simulink model "sraam2023b"  (R2023b)
settings: Solver=ode4  StartTime=0.0  StopTime=25  FixedStep=0.001  RelTol=1e-3
values from neighbouring files (symbols this model uses):
  AEXIT = 0.0125    [SRAAM6_params.m]
  ALIMIT = 50.0    (= 50)    [SRAAM6_params.m]
  ALP_LIMX = 46.0    (= 46)    [SRAAM6_params.m]
  BIASAL = 0.0    (= 0)    [SRAAM6_params.m]
  DDLIMX = 600.0    (= 600)    [SRAAM6_params.m]
  DLIMX = 28.0    (= 28)    [SRAAM6_params.m]
  DPLIMX = 28.0    (= 28)    [SRAAM6_params.m]
  DQLIMX = 28.0    (= 28)    [SRAAM6_params.m]
  DRLIMX = 28.0    (= 28)    [SRAAM6_params.m]
  DT = 0.001    [SRAAM6_params.m]
  EBIASA = zeros(3,1)    [SRAAM6_params.m]
  EBIASG = zeros(3,1)    [SRAAM6_params.m]
  EMISA = zeros(3,1)    [SRAAM6_params.m]
  EMISG = zeros(3,1)    [SRAAM6_params.m]
  ESCALA = zeros(3,1)    [SRAAM6_params.m]
  ESCALG = zeros(3,1)    [SRAAM6_params.m]
  EUNBG = zeros(3,1)    [SRAAM6_params.m]
  FACT_WRCL = 0.0    (= 0)    [SRAAM6_params.m]
  GNAV = 4.0    (= 4)    [SRAAM6_params.m]
  INS_NOISE_PWR_A = 0.0    (= 0)    [SRAAM6_params.m]
  INS_NOISE_PWR_G = 0.0    (= 0)    [SRAAM6_params.m]
  K_ALPHA = 10.0    (= 10)    [SRAAM6_params.m]
  K_BETA = 10.0    (= 10)    [SRAAM6_params.m]
  MINS = 0    [SRAAM6_params.m]
  prop_cg_t = prop_cg_vs_time_t(:)    [SRAAM6_params.m]
  prop_cg_v = prop_cg_vs_time_v(:)    [SRAAM6_params.m]
  prop_mass_t = prop_mass_vs_time_t(:)    [SRAAM6_params.m]
  prop_mass_v = prop_mass_vs_time_v(:)    [SRAAM6_params.m]
  prop_moipitch_t = prop_moipitch_vs_time_t(:)    [SRAAM6_params.m]
  prop_moipitch_v = prop_moipitch_vs_time_v(:)    [SRAAM6_params.m]
  prop_moiroll_t = prop_moiroll_vs_time_t(:)    [SRAAM6_params.m]
  prop_moiroll_v = prop_moiroll_vs_time_v(:)    [SRAAM6_params.m]
  prop_thrust_t = prop_thrust_vs_time_t(:)    [SRAAM6_params.m]
  prop_thrust_v = prop_thrust_vs_time_v(:)    [SRAAM6_params.m]
  REFA = 0.01824    [SRAAM6_params.m]
  REFL = 0.1524    [SRAAM6_params.m]
  SCENARIO = 12    [SRAAM6_params.m]
  TGET_POS_IC = TGET_POS(SCENARIO, :)'    [SRAAM6_params.m]
  TGET_VEL_IC = TGET_VEL(SCENARIO, :)'    [SRAAM6_params.m]
  WBLIMX = 30.0    (= 30)    [SRAAM6_params.m]
  WN_NDI_Q = 50.0    (= 50)    [SRAAM6_params.m]
  WN_NDI_R = 50.0    (= 50)    [SRAAM6_params.m]
  WNACT = 251.0    (= 251)    [SRAAM6_params.m]
  X_IC = [SBEL_INIT; VBEB_IC; Q_IC; OMEGA_IC]    [SRAAM6_params.m]
  XCG_REF = 1.2994    [SRAAM6_params.m]
  ZETACT = 0.7    [SRAAM6_params.m]
  ZRCL = 0.9    [SRAAM6_params.m]
undefined symbols (not defined in the file or in its folder): alpha_bp, beta_bp, ca0_vs_mach, ca0b_vs_mach, caa_vs_mach_alpha_beta, cad_vs_mach, cll0_vs_mach_alpha_beta, clldp_vs_mach_alpha_beta, cllp_vs_mach, clm0_vs_mach_alpha_beta, clmdq_vs_mach_alpha_beta, clmq_vs_mach, cln0_vs_mach_alpha_beta, clndr_vs_mach_alpha_beta, clnr_vs_mach, cn0_vs_mach_alpha_beta, cndq_vs_mach_alpha_beta, cy0_vs_mach_alpha_beta, cydr_vs_mach_alpha_beta, mach_bp
libraries: simulink x3
(part 1 of 2)
settings Model: Creator=yagiz  LastModifiedBy=yagiz
settings DataIOCC: SaveFormat=Array  SaveState=on
settings RTWCC: GPUComputeCapability=5.0

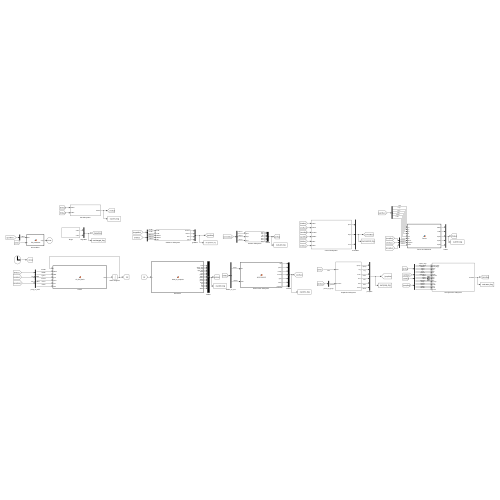
[thumbnail: Simulink's stored preview of the top-level diagram]
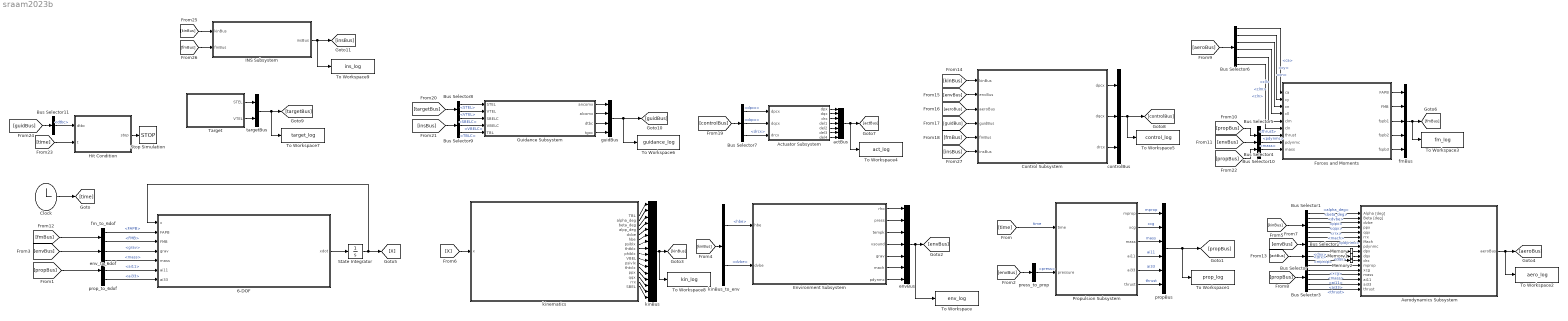
== system sraam2023b ==
  6-DOF : MATLAB Function  TreatAsAtomicUnit=on
  Actuator Subsystem : Subsystem
  Aerodynamics Subsystem : Subsystem
  Bus Selector : BusSelector  OutputSignals=dpx,dqx,drx
  Bus Selector1 : BusSelector  OutputSignals=alpha_deg,beta_deg,dvbe,ppx,qqx,rrx
  Bus Selector10 : BusSelector  OutputSignals=mass
  Bus Selector11 : BusSelector  OutputSignals=dtbc
  Bus Selector2 : BusSelector  OutputSignals=mach,pdynmc
  Bus Selector3 : BusSelector  OutputSignals=mprop,xcg,mass,ai11,ai33,thrust
  Bus Selector4 : BusSelector  OutputSignals=pdynmc
  Bus Selector5 : BusSelector  OutputSignals=thrust
  Bus Selector6 : BusSelector  OutputSignals=ca,cy,cn,cll,clm,cln
  Bus Selector7 : BusSelector  OutputSignals=dpcx,dqcx,drcx
  Bus Selector8 : BusSelector  OutputSignals=STEL,VTEL
  Bus Selector9 : BusSelector  OutputSignals=SBELC,VBELC,TBLC
  Clock : Clock
  Control Subsystem : Subsystem
  Environment Subsystem : MATLAB Function  TreatAsAtomicUnit=on
  Forces and Moments : MATLAB Function  TreatAsAtomicUnit=on
  Guidance Subsystem : Subsystem
  Hit Condition : MATLAB Function  TreatAsAtomicUnit=on
  INS Subsystem : Subsystem
  Memory : Memory
  Memory1 : Memory
  Memory2 : Memory
  Propulsion Subsystem : Subsystem
  State Integrator : Integrator  InitialCondition=X_IC
  Stop Simulation : Stop
  Target : Subsystem
  To Workspace : ToWorkspace  VariableName=env_log  SaveFormat=Timeseries  SampleTime=-1
  To Workspace1 : ToWorkspace  VariableName=prop_log  SaveFormat=Timeseries  SampleTime=-1
  To Workspace2 : ToWorkspace  VariableName=aero_log  SaveFormat=Timeseries  SampleTime=-1
  To Workspace3 : ToWorkspace  VariableName=fm_log  SaveFormat=Timeseries  SampleTime=-1
  To Workspace4 : ToWorkspace  VariableName=act_log  SaveFormat=Timeseries  SampleTime=-1
  To Workspace5 : ToWorkspace  VariableName=control_log  SaveFormat=Timeseries  SampleTime=-1
  To Workspace6 : ToWorkspace  VariableName=guidance_log  SaveFormat=Timeseries  SampleTime=-1
  To Workspace7 : ToWorkspace  VariableName=target_log  SaveFormat=Timeseries  SampleTime=-1
  To Workspace8 : ToWorkspace  VariableName=kin_log  SaveFormat=Timeseries  SampleTime=-1
  To Workspace9 : ToWorkspace  VariableName=ins_log  SaveFormat=Timeseries  SampleTime=-1
  actBus : BusCreator  Inputs=7
  controlBus : BusCreator  Inputs=3
  envBus : BusCreator  Inputs=7
  env_to_6dof : BusSelector  OutputSignals=grav
  fmBus : BusCreator  Inputs=5
  fm_to_6dof : BusSelector  OutputSignals=FAPB,FMB
  guidBus : BusCreator  Inputs=4
  kinBus : BusCreator  Inputs=16
  kinBus_to_env : BusSelector  OutputSignals=hbe,dvbe
  kinematics : MATLAB Function  TreatAsAtomicUnit=on
  press_to_prop : BusSelector  OutputSignals=press
  propBus : BusCreator  Inputs=6
  prop_to_6dof : BusSelector  OutputSignals=mass,ai11,ai33
  targetBus : BusCreator  Inputs=2
  wires:
  6-DOF/1(xdot) -> State Integrator/1
  State Integrator/1 -> [X], 6-DOF/1(x)
  Clock/1 -> [time]
  Environment Subsystem/7(pdynmc) -> envBus/7
  Environment Subsystem/6(mach) -> envBus/6
  Environment Subsystem/5(grav) -> envBus/5
  Environment Subsystem/4(vsound) -> envBus/4
  Environment Subsystem/3(tempk) -> envBus/3
  Environment Subsystem/2(press) -> envBus/2
  Environment Subsystem/1(rho) -> envBus/1
  envBus/1 -> To Workspace/1, [envBus]
  press_to_prop/1 -> Propulsion Subsystem/2(pressure)  "<press>"
  [time] -> Propulsion Subsystem/1(time)  "time"
  Propulsion Subsystem/1(mprop) -> propBus/1  "mprop"
  Propulsion Subsystem/2(xcg) -> propBus/2  "xcg"
  Propulsion Subsystem/3(mass) -> propBus/3  "mass"
  Propulsion Subsystem/4(ai11) -> propBus/4  "ai11"
  Propulsion Subsystem/5(ai33) -> propBus/5  "ai33"
  Propulsion Subsystem/6(thrust) -> propBus/6  "thrust"
  propBus/1 -> [propBus], To Workspace1/1
  [propBus] -> prop_to_6dof/1
  prop_to_6dof/1 -> 6-DOF/5(mass)  "<mass>"
  prop_to_6dof/2 -> 6-DOF/6(ai11)  "<ai11>"
  prop_to_6dof/3 -> 6-DOF/7(ai33)  "<ai33>"
  [envBus] -> press_to_prop/1
  [envBus] -> env_to_6dof/1
  env_to_6dof/1 -> 6-DOF/4(grav)  "<grav>"
  [X] -> kinematics/1(x)
  Aerodynamics Subsystem/1(aeroBus) -> To Workspace2/1, [aeroBus]
  kinematics/1(TBL) -> kinBus/1
  kinematics/2(alpha_deg) -> kinBus/2
  kinematics/3(beta_deg) -> kinBus/3
  kinematics/4(alpp_deg) -> kinBus/4
  kinematics/5(dvbe) -> kinBus/5
  kinematics/6(hbe) -> kinBus/6
  kinematics/7(psiblx) -> kinBus/7
  kinematics/8(thtblx) -> kinBus/8
  kinematics/9(phiblx) -> kinBus/9
  kinematics/10(VBEL) -> kinBus/10
  kinematics/11(psivlx) -> kinBus/11
  kinematics/12(thtvlx) -> kinBus/12
  kinBus/1 -> To Workspace8/1, [kinBus]
  [kinBus] -> kinBus_to_env/1
  kinBus_to_env/1 -> Environment Subsystem/1(hbe)  "<hbe>"
  kinBus_to_env/2 -> Environment Subsystem/2(dvbe)  "<dvbe>"
  [kinBus] -> Bus Selector1/1
  Bus Selector1/1 -> Aerodynamics Subsystem/1(Alpha [deg])  "<alpha_deg>"
  Bus Selector1/2 -> Aerodynamics Subsystem/2(Beta [deg])  "<beta_deg>"
  Bus Selector1/3 -> Aerodynamics Subsystem/3(dvbe)  "<dvbe>"
  Bus Selector1/4 -> Aerodynamics Subsystem/4(ppx)  "<ppx>"
  Bus Selector1/5 -> Aerodynamics Subsystem/5(qqx)  "<qqx>"
  Bus Selector1/6 -> Aerodynamics Subsystem/6(rrx)  "<rrx>"
  [envBus] -> Bus Selector2/1
  Bus Selector2/1 -> Aerodynamics Subsystem/7(Mach)  "<mach>"
  Bus Selector2/2 -> Aerodynamics Subsystem/8(pdynmc)  "<pdynmc>"
  [propBus] -> Bus Selector3/1
  Bus Selector3/1 -> Aerodynamics Subsystem/12(mprop)  "<mprop>"
  Bus Selector3/2 -> Aerodynamics Subsystem/13(xcg)  "<xcg>"
  Bus Selector3/3 -> Aerodynamics Subsystem/14(mass)  "<mass>"
  Bus Selector3/4 -> Aerodynamics Subsystem/15(ai11)  "<ai11>"
  Bus Selector3/5 -> Aerodynamics Subsystem/16(ai33)  "<ai33>"
  Bus Selector3/6 -> Aerodynamics Subsystem/17(thrust)  "<thrust>"
  [envBus] -> Bus Selector4/1
  Bus Selector4/1 -> Forces and Moments/8(pdynmc)  "<pdynmc>"
  [propBus] -> Bus Selector5/1
  [aeroBus] -> Bus Selector6/1
  Bus Selector6/1 -> Forces and Moments/1(ca)  "<ca>"
  Bus Selector6/2 -> Forces and Moments/2(cy)  "<cy>"
  Bus Selector6/3 -> Forces and Moments/3(cn)  "<cn>"
  Bus Selector6/4 -> Forces and Moments/4(cll)  "<cll>"
  Bus Selector6/5 -> Forces and Moments/5(clm)  "<clm>"
  Bus Selector6/6 -> Forces and Moments/6(cln)  "<cln>"
  Bus Selector5/1 -> Forces and Moments/7(thrust)  "<thrust>"
  Forces and Moments/1(FAPB) -> fmBus/1
  Forces and Moments/2(FMB) -> fmBus/2
  [fmBus] -> fm_to_6dof/1
  fm_to_6dof/1 -> 6-DOF/2(FAPB)  "<FAPB>"
  fm_to_6dof/2 -> 6-DOF/3(FMB)  "<FMB>"
  Actuator Subsystem/1(dpx) -> actBus/1
  Actuator Subsystem/2(dqx) -> actBus/2
  Actuator Subsystem/3(drx) -> actBus/3
  Actuator Subsystem/4(del1) -> actBus/4
  Actuator Subsystem/5(del2) -> actBus/5
  Actuator Subsystem/6(del3) -> actBus/6
  Actuator Subsystem/7(del4) -> actBus/7
  actBus/1 -> To Workspace4/1, [actBus]
  [actBus] -> Bus Selector/1
  Bus Selector/1 -> Memory/1  "<dpx>"
  Bus Selector/2 -> Memory1/1  "<dqx>"
  Bus Selector/3 -> Memory2/1  "<drx>"
  [kinBus] -> Control Subsystem/1(kinBus)
  [envBus] -> Control Subsystem/2(envBus)
  [aeroBus] -> Control Subsystem/3(aeroBus)
  controlBus/1 -> To Workspace5/1, [controlBus]
  [controlBus] -> Bus Selector7/1
  Bus Selector7/2 -> Actuator Subsystem/2(dqcx)  "<dqcx>"
  Bus Selector7/3 -> Actuator Subsystem/3(drcx)  "<drcx>"
  Bus Selector7/1 -> Actuator Subsystem/1(dpcx)  "<dpcx>"
  Control Subsystem/1(dpcx) -> controlBus/1
  Memory/1 -> Aerodynamics Subsystem/9(dpx)
  Memory1/1 -> Aerodynamics Subsystem/10(dqx)
  Memory2/1 -> Aerodynamics Subsystem/11(drx)
  Target/1(STEL) -> targetBus/1
  Target/2(VTEL) -> targetBus/2
  targetBus/1 -> To Workspace7/1, [targetBus]
  [targetBus] -> Bus Selector8/1
  Bus Selector8/1 -> Guidance Subsystem/1(STEL)  "<STEL>"
  Bus Selector8/2 -> Guidance Subsystem/2(VTEL)  "<VTEL>"
  [insBus] -> Bus Selector9/1
  Guidance Subsystem/1(ancomx) -> guidBus/1
  Guidance Subsystem/2(alcomx) -> guidBus/2
  guidBus/1 -> To Workspace6/1, [guidBus]
  [guidBus] -> Control Subsystem/4(guidBus)
  [propBus] -> Bus Selector10/1
  Bus Selector10/1 -> Forces and Moments/9(mass)  "<mass>"
  fmBus/1 -> [fmBus], To Workspace3/1
  [fmBus] -> Control Subsystem/5(fmBus)
  Guidance Subsystem/3(dtbc) -> guidBus/3
  Guidance Subsystem/4(tgoc) -> guidBus/4
  [time] -> Hit Condition/2(t)
  [guidBus] -> Bus Selector11/1
  Bus Selector11/1 -> Hit Condition/1(dtbc)  "<dtbc>"
  Hit Condition/1(stop) -> Stop Simulation/1
  Control Subsystem/2(dqcx) -> controlBus/2
  Control Subsystem/3(drcx) -> controlBus/3
  kinematics/13(ppx) -> kinBus/13
  kinematics/14(qqx) -> kinBus/14
  kinematics/15(rrx) -> kinBus/15
  kinematics/16(SBEL) -> kinBus/16
  Forces and Moments/3(fspb1) -> fmBus/3
  Forces and Moments/4(fspb2) -> fmBus/4
  Forces and Moments/5(fspb3) -> fmBus/5
  [kinBus] -> INS Subsystem/1(kinBus)
  [fmBus] -> INS Subsystem/2(fmBus)
  INS Subsystem/1(insBus) -> To Workspace9/1, [insBus]
  Bus Selector9/1 -> Guidance Subsystem/3(SBELC)  "<SBELC>"
  Bus Selector9/2 -> Guidance Subsystem/4(VBELC)  "<VBELC>"
  Bus Selector9/3 -> Guidance Subsystem/5(TBL)  "<TBLC>"
  [insBus] -> Control Subsystem/6(insBus)

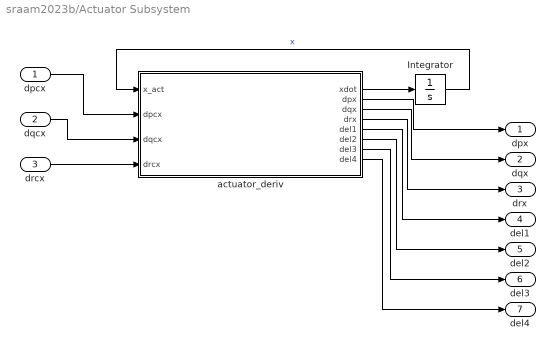
== system sraam2023b/Actuator Subsystem ==
  dpcx : Inport
  dqcx : Inport  Port=2
  drcx : Inport  Port=3
  Integrator : Integrator  InitialCondition=zeros(8, 1)
  actuator_deriv : MATLAB Function  TreatAsAtomicUnit=on
  dpx : Outport
  dqx : Outport  Port=2
  drx : Outport  Port=3
  del1 : Outport  Port=4
  del2 : Outport  Port=5
  del3 : Outport  Port=6
  del4 : Outport  Port=7
  wires:
  actuator_deriv/1(xdot) -> Integrator/1
  Integrator/1 -> actuator_deriv/1(x_act)  "x"
  dpcx/1 -> actuator_deriv/2(dpcx)
  dqcx/1 -> actuator_deriv/3(dqcx)
  drcx/1 -> actuator_deriv/4(drcx)
  actuator_deriv/2(dpx) -> dpx/1
  actuator_deriv/3(dqx) -> dqx/1
  actuator_deriv/4(drx) -> drx/1
  actuator_deriv/5(del1) -> del1/1
  actuator_deriv/6(del2) -> del2/1
  actuator_deriv/7(del3) -> del3/1
  actuator_deriv/8(del4) -> del4/1

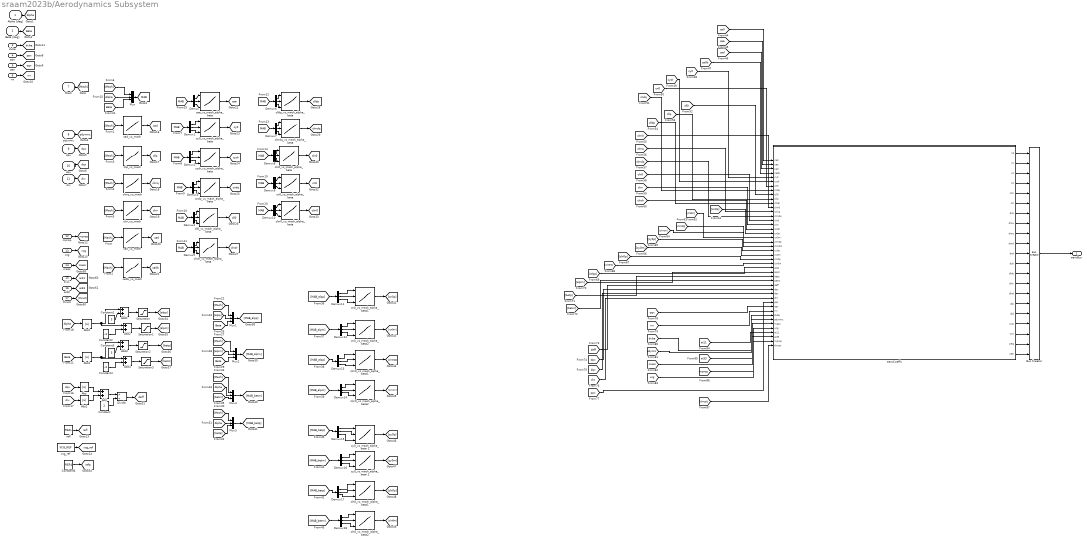
== system sraam2023b/Aerodynamics Subsystem ==
  Alpha [deg] : Inport
  Beta [deg] : Inport  Port=2
  dvbe : Inport  Port=3
  ppx : Inport  Port=4
  qqx : Inport  Port=5
  rrx : Inport  Port=6
  Mach : Inport  Port=7
  pdynmc : Inport  Port=8
  dpx : Inport  Port=9
  dqx : Inport  Port=10
  drx : Inport  Port=11
  mprop : Inport  Port=12
  xcg : Inport  Port=13
  mass : Inport  Port=14
  ai11 : Inport  Port=15
  ai33 : Inport  Port=16
  thrust : Inport  Port=17
  Abs{,1..3} (4 alike) : Abs  SaturateOnIntegerOverflow=off
  Add{,1..4} (5 alike) : Sum
  Bus Creator : BusCreator  Inputs=21
  Constant : Constant  Value=2
  Constant1 : Constant  Value=3
  Constant2 : Constant  Value=-3
  Constant3 : Constant  Value=3
  Constant4 : Constant  Value=-3
  Constant6 : Constant  Value=REFA
  Demux{,1..18} (19 alike) : Demux  Outputs=3
  Divide : Product  Inputs=*/
  Mux{,1..4} (5 alike) : Mux  Inputs=3
  Saturation : Saturate  UpperLimit=inf  LowerLimit=3
  Saturation1 : Saturate  UpperLimit=inf  LowerLimit=0
  Saturation2 : Saturate  UpperLimit=inf  LowerLimit=3
  Saturation3 : Saturate  UpperLimit=inf  LowerLimit=0
  aeroCoeffs : MATLAB Function  TreatAsAtomicUnit=on
  ca0_vs_mach : Lookup_n-D  NumberOfTableDimensions=1  BreakpointsForDimension1=mach_bp  Table=ca0_vs_mach  InternalRulePriority=Speed  RndMeth=Simplest
  ca0b_vs_mach : Lookup_n-D  NumberOfTableDimensions=1  BreakpointsForDimension1=mach_bp  Table=ca0b_vs_mach  InternalRulePriority=Speed  RndMeth=Simplest
  caa_vs_mach_alpha_beta : Lookup_n-D  NumberOfTableDimensions=3  BreakpointsForDimension1=mach_bp  BreakpointsForDimension2=alpha_bp  BreakpointsForDimension3=beta_bp  Table=caa_vs_mach_alpha_beta  InternalRulePriority=Speed  RndMeth=Simplest
      settings: InputPortMap=u0,u1,u2
  cad_vs_mach : Lookup_n-D  NumberOfTableDimensions=1  BreakpointsForDimension1=mach_bp  Table=cad_vs_mach  InternalRulePriority=Speed  RndMeth=Simplest
  cll0_vs_mach_alpha_beta : Lookup_n-D  NumberOfTableDimensions=3  BreakpointsForDimension1=mach_bp  BreakpointsForDimension2=alpha_bp  BreakpointsForDimension3=beta_bp  Table=cll0_vs_mach_alpha_beta  InternalRulePriority=Speed  RndMeth=Simplest
      settings: InputPortMap=u0,u1,u2
  clldp_vs_mach_alpha_beta : Lookup_n-D  NumberOfTableDimensions=3  BreakpointsForDimension1=mach_bp  BreakpointsForDimension2=alpha_bp  BreakpointsForDimension3=beta_bp  Table=clldp_vs_mach_alpha_beta  InternalRulePriority=Speed  RndMeth=Simplest
      settings: InputPortMap=u0,u1,u2
  cllp_vs_mach : Lookup_n-D  NumberOfTableDimensions=1  BreakpointsForDimension1=mach_bp  Table=cllp_vs_mach  InternalRulePriority=Speed  RndMeth=Simplest
  clm0_vs_mach_alpha_beta : Lookup_n-D  NumberOfTableDimensions=3  BreakpointsForDimension1=mach_bp  BreakpointsForDimension2=alpha_bp  BreakpointsForDimension3=beta_bp  Table=clm0_vs_mach_alpha_beta  InternalRulePriority=Speed  RndMeth=Simplest
      settings: InputPortMap=u0,u1,u2
  clm0_vs_mach_alpha_beta1 : Lookup_n-D  NumberOfTableDimensions=3  BreakpointsForDimension1=mach_bp  BreakpointsForDimension2=alpha_bp  BreakpointsForDimension3=beta_bp  Table=clm0_vs_mach_alpha_beta  InternalRulePriority=Speed  RndMeth=Simplest
      settings: InputPortMap=u0,u1,u2
  clm0_vs_mach_alpha_beta2 : Lookup_n-D  NumberOfTableDimensions=3  BreakpointsForDimension1=mach_bp  BreakpointsForDimension2=alpha_bp  BreakpointsForDimension3=beta_bp  Table=clm0_vs_mach_alpha_beta  InternalRulePriority=Speed  RndMeth=Simplest
      settings: InputPortMap=u0,u1,u2
  clmdq_vs_mach_alpha_beta : Lookup_n-D  NumberOfTableDimensions=3  BreakpointsForDimension1=mach_bp  BreakpointsForDimension2=alpha_bp  BreakpointsForDimension3=beta_bp  Table=clmdq_vs_mach_alpha_beta  InternalRulePriority=Speed  RndMeth=Simplest
      settings: InputPortMap=u0,u1,u2
  clmq_vs_mach : Lookup_n-D  NumberOfTableDimensions=1  BreakpointsForDimension1=mach_bp  Table=clmq_vs_mach  InternalRulePriority=Speed  RndMeth=Simplest
  cln0_vs_mach_alpha_beta : Lookup_n-D  NumberOfTableDimensions=3  BreakpointsForDimension1=mach_bp  BreakpointsForDimension2=alpha_bp  BreakpointsForDimension3=beta_bp  Table=cln0_vs_mach_alpha_beta  InternalRulePriority=Speed  RndMeth=Simplest
      settings: InputPortMap=u0,u1,u2
  cln0_vs_mach_alpha_beta1 : Lookup_n-D  NumberOfTableDimensions=3  BreakpointsForDimension1=mach_bp  BreakpointsForDimension2=alpha_bp  BreakpointsForDimension3=beta_bp  Table=cln0_vs_mach_alpha_beta  InternalRulePriority=Speed  RndMeth=Simplest
      settings: InputPortMap=u0,u1,u2
  cln0_vs_mach_alpha_beta2 : Lookup_n-D  NumberOfTableDimensions=3  BreakpointsForDimension1=mach_bp  BreakpointsForDimension2=alpha_bp  BreakpointsForDimension3=beta_bp  Table=cln0_vs_mach_alpha_beta  InternalRulePriority=Speed  RndMeth=Simplest
      settings: InputPortMap=u0,u1,u2
  "clndr_vs_mach_alpha_beta " : Lookup_n-D  NumberOfTableDimensions=3  BreakpointsForDimension1=mach_bp  BreakpointsForDimension2=alpha_bp  BreakpointsForDimension3=beta_bp  Table=clndr_vs_mach_alpha_beta  InternalRulePriority=Speed  RndMeth=Simplest
      settings: InputPortMap=u0,u1,u2
  clnr_vs_mach : Lookup_n-D  NumberOfTableDimensions=1  BreakpointsForDimension1=mach_bp  Table=clnr_vs_mach  InternalRulePriority=Speed  RndMeth=Simplest
  cn0_vs_mach_alpha_beta : Lookup_n-D  NumberOfTableDimensions=3  BreakpointsForDimension1=mach_bp  BreakpointsForDimension2=alpha_bp  BreakpointsForDimension3=beta_bp  Table=cn0_vs_mach_alpha_beta  InternalRulePriority=Speed  RndMeth=Simplest
      settings: InputPortMap=u0,u1,u2
  cn0_vs_mach_alpha_beta1 : Lookup_n-D  NumberOfTableDimensions=3  BreakpointsForDimension1=mach_bp  BreakpointsForDimension2=alpha_bp  BreakpointsForDimension3=beta_bp  Table=cn0_vs_mach_alpha_beta  InternalRulePriority=Speed  RndMeth=Simplest
      settings: InputPortMap=u0,u1,u2
  cn0_vs_mach_alpha_beta2 : Lookup_n-D  NumberOfTableDimensions=3  BreakpointsForDimension1=mach_bp  BreakpointsForDimension2=alpha_bp  BreakpointsForDimension3=beta_bp  Table=cn0_vs_mach_alpha_beta  InternalRulePriority=Speed  RndMeth=Simplest
      settings: InputPortMap=u0,u1,u2
  cndq_vs_mach_alpha_beta : Lookup_n-D  NumberOfTableDimensions=3  BreakpointsForDimension1=mach_bp  BreakpointsForDimension2=alpha_bp  BreakpointsForDimension3=beta_bp  Table=cndq_vs_mach_alpha_beta  InternalRulePriority=Speed  RndMeth=Simplest
      settings: InputPortMap=u0,u1,u2
  "cy0_vs_mach_alpha_beta " : Lookup_n-D  NumberOfTableDimensions=3  BreakpointsForDimension1=mach_bp  BreakpointsForDimension2=alpha_bp  BreakpointsForDimension3=beta_bp  Table=cy0_vs_mach_alpha_beta  InternalRulePriority=Speed  RndMeth=Simplest
      settings: InputPortMap=u0,u1,u2
  cy0_vs_mach_alpha_beta 1 : Lookup_n-D  NumberOfTableDimensions=3  BreakpointsForDimension1=mach_bp  BreakpointsForDimension2=alpha_bp  BreakpointsForDimension3=beta_bp  Table=cy0_vs_mach_alpha_beta  InternalRulePriority=Speed  RndMeth=Simplest
      settings: InputPortMap=u0,u1,u2
  cy0_vs_mach_alpha_beta 2 : Lookup_n-D  NumberOfTableDimensions=3  BreakpointsForDimension1=mach_bp  BreakpointsForDimension2=alpha_bp  BreakpointsForDimension3=beta_bp  Table=cy0_vs_mach_alpha_beta  InternalRulePriority=Speed  RndMeth=Simplest
      settings: InputPortMap=u0,u1,u2
  cydr_vs_mach_alpha_beta : Lookup_n-D  NumberOfTableDimensions=3  BreakpointsForDimension1=mach_bp  BreakpointsForDimension2=alpha_bp  BreakpointsForDimension3=beta_bp  Table=cydr_vs_mach_alpha_beta  InternalRulePriority=Speed  RndMeth=Simplest
      settings: InputPortMap=u0,u1,u2
  refl : Constant  Value=REFL
  xcg_ref : Constant  Value=XCG_REF
  aeroBus : Outport
  tag scope: Alpha=global, Beta=global, MAB=global, ai11=global, ai33=global, ca0=global, ca0b=global, caa=global, cad=global, cll0=global, clldp=global, cllp=global, clm0=global, clmdq=global, clmq=global, cln0=global, clndr=global, clnr=global, cn0=global, cndq=global, cy0=global, cydr=global, deff=global, dpx=global, dqx=global, drx=global, dvbe=global, mass=global, mprop=global, pdynmc=global, ppx=global, qqx=global, refa=global, refl=global, rrx=global, xcg=global, xcg_ref=global
  wires:
  Demux7/2 -> clmdq_vs_mach_alpha_beta/2
  [drx] -> Abs1/1
  [Mach] -> Mux/1
  Demux5/1 -> "clndr_vs_mach_alpha_beta "/1
  Demux7/3 -> clmdq_vs_mach_alpha_beta/3
  caa_vs_mach_alpha_beta/1 -> [caa]
  Demux9/3 -> cn0_vs_mach_alpha_beta/3
  Demux2/1 -> cydr_vs_mach_alpha_beta/1
  Demux/2 -> caa_vs_mach_alpha_beta/2
  Demux4/1 -> cll0_vs_mach_alpha_beta/1
  [MAB] -> Demux5/1
  [Mach] -> cad_vs_mach/1
  [MAB] -> Demux6/1
  Alpha [deg]/1 -> [Alpha]
  dqx/1 -> [dqx]
  [MAB] -> Demux4/1
  [MAB] -> Demux8/1
  Mux/1 -> [MAB]
  Demux1/1 -> "cy0_vs_mach_alpha_beta "/1
  Divide/1 -> [deff]
  clm0_vs_mach_alpha_beta/1 -> [clm0]
  cllp_vs_mach/1 -> [cllp]
  [Mach] -> clnr_vs_mach/1
  [MAB] -> Demux9/1
  Demux8/1 -> cln0_vs_mach_alpha_beta/1
  Add/1 -> Divide/1
  drx/1 -> [drx]
  Demux/3 -> caa_vs_mach_alpha_beta/3
  Mach/1 -> [Mach]
  Demux2/3 -> cydr_vs_mach_alpha_beta/3
  clmq_vs_mach/1 -> [clmq]
  Abs/1 -> Add/1
  clmdq_vs_mach_alpha_beta/1 -> [clmdq]
  Demux6/3 -> clldp_vs_mach_alpha_beta/3
  Beta [deg]/1 -> [Beta]
  Demux8/2 -> cln0_vs_mach_alpha_beta/2
  cndq_vs_mach_alpha_beta/1 -> [cndq]
  Demux2/2 -> cydr_vs_mach_alpha_beta/2
  Demux9/1 -> cn0_vs_mach_alpha_beta/1
  Demux3/3 -> cndq_vs_mach_alpha_beta/3
  Demux7/1 -> clmdq_vs_mach_alpha_beta/1
  Demux10/1 -> clm0_vs_mach_alpha_beta/1
  Demux1/2 -> "cy0_vs_mach_alpha_beta "/2
  Demux5/2 -> "clndr_vs_mach_alpha_beta "/2
  cn0_vs_mach_alpha_beta/1 -> [cn0]
  ca0b_vs_mach/1 -> [ca0b]
  Demux3/1 -> cndq_vs_mach_alpha_beta/1
  [Alpha] -> Mux/2
  [Mach] -> ca0_vs_mach/1
  clldp_vs_mach_alpha_beta/1 -> [clldp]
  Constant/1 -> Divide/2
  [dqx] -> Abs/1
  ai33/1 -> [ai33]
  Demux5/3 -> "clndr_vs_mach_alpha_beta "/3
  [MAB] -> Demux10/1
  [MAB] -> Demux2/1
  Demux6/1 -> clldp_vs_mach_alpha_beta/1
  Demux8/3 -> cln0_vs_mach_alpha_beta/3
  "clndr_vs_mach_alpha_beta "/1 -> [clndr]
  pdynmc/1 -> [pdynmc]
  dpx/1 -> [dpx]
  xcg/1 -> [xcg]
  Demux1/3 -> "cy0_vs_mach_alpha_beta "/3
  [Mach] -> ca0b_vs_mach/1
  [MAB] -> Demux3/1
  Abs1/1 -> Add/2
  [Mach] -> cllp_vs_mach/1
  Demux3/2 -> cndq_vs_mach_alpha_beta/2
  [MAB] -> Demux1/1
  cydr_vs_mach_alpha_beta/1 -> [cydr]
  Demux4/2 -> cll0_vs_mach_alpha_beta/2
  Demux/1 -> caa_vs_mach_alpha_beta/1
  mprop/1 -> [mprop]
  Demux9/2 -> cn0_vs_mach_alpha_beta/2
  [Mach] -> clmq_vs_mach/1
  cad_vs_mach/1 -> [cad]
  Demux10/2 -> clm0_vs_mach_alpha_beta/2
  [Beta] -> Mux/3
  Demux6/2 -> clldp_vs_mach_alpha_beta/2
  ca0_vs_mach/1 -> [ca0]
  clnr_vs_mach/1 -> [clnr]
  [MAB] -> Demux7/1
  "cy0_vs_mach_alpha_beta "/1 -> [cy0]
  mass/1 -> [mass]
  cll0_vs_mach_alpha_beta/1 -> [cll0]
  ai11/1 -> [ai11]
  cln0_vs_mach_alpha_beta/1 -> [cln0]
  Demux4/3 -> cll0_vs_mach_alpha_beta/3
  Demux10/3 -> clm0_vs_mach_alpha_beta/3
  [MAB] -> Demux/1
  Add2/1 -> Saturation1/1
  Saturation2/1 -> [betp]
  Constant3/1 -> Add3/2
  [Beta] -> Abs3/1
  Abs2/1 -> Add2/1, Add1/1
  Constant2/1 -> Add2/2
  Constant4/1 -> Add4/2
  Saturation3/1 -> [betm]
  Add1/1 -> Saturation/1
  Saturation/1 -> [alpp]
  Constant1/1 -> Add1/2
  Add3/1 -> Saturation2/1
  [Alpha] -> Abs2/1
  Saturation1/1 -> [alpm]
  Abs3/1 -> Add4/1, Add3/1
  Add4/1 -> Saturation3/1
  refl/1 -> [refl]
  Constant6/1 -> [refa]
  xcg_ref/1 -> [xcg_ref]
  [Beta] -> Mux2/3
  [Mach] -> Mux2/1
  [Beta] -> Mux1/3
  [Alpha] -> Mux3/2
  Mux3/1 -> [MAB_betp]
  [betm] -> Mux4/3
  [Mach] -> Mux3/1
  [betp] -> Mux3/3
  Mux1/1 -> [MAB_alpp]
  [alpm] -> Mux2/2
  [Mach] -> Mux1/1
  [alpp] -> Mux1/2
  [Mach] -> Mux4/1
  [Alpha] -> Mux4/2
  Mux2/1 -> [MAB_alpm]
  Mux4/1 -> [MAB_betm]
  Demux18/2 -> cln0_vs_mach_alpha_beta2/2
  cy0_vs_mach_alpha_beta 2/1 -> [cy0m]
  Demux13/3 -> clm0_vs_mach_alpha_beta1/3
  clm0_vs_mach_alpha_beta1/1 -> [clm0p]
  cln0_vs_mach_alpha_beta2/1 -> [cln0m]
  [MAB_alpp] -> Demux11/1
  [MAB_betm] -> Demux18/1
  Demux11/1 -> cn0_vs_mach_alpha_beta1/1
  Demux14/1 -> clm0_vs_mach_alpha_beta2/1
  Demux12/3 -> cn0_vs_mach_alpha_beta2/3
  Demux17/3 -> cln0_vs_mach_alpha_beta1/3
  Demux14/3 -> clm0_vs_mach_alpha_beta2/3
  cy0_vs_mach_alpha_beta 1/1 -> [cy0p]
  [MAB_betp] -> Demux17/1
  Demux11/3 -> cn0_vs_mach_alpha_beta1/3
  Demux16/3 -> cy0_vs_mach_alpha_beta 2/3
  Demux15/3 -> cy0_vs_mach_alpha_beta 1/3
  [MAB_betm] -> Demux16/1
  Demux11/2 -> cn0_vs_mach_alpha_beta1/2
  [MAB_betp] -> Demux15/1
  Demux15/1 -> cy0_vs_mach_alpha_beta 1/1
  Demux14/2 -> clm0_vs_mach_alpha_beta2/2
  cn0_vs_mach_alpha_beta1/1 -> [cn0p]
  Demux16/1 -> cy0_vs_mach_alpha_beta 2/1
  Demux13/2 -> clm0_vs_mach_alpha_beta1/2
  Demux17/1 -> cln0_vs_mach_alpha_beta1/1
  Demux12/2 -> cn0_vs_mach_alpha_beta2/2
  Demux12/1 -> cn0_vs_mach_alpha_beta2/1
  Demux15/2 -> cy0_vs_mach_alpha_beta 1/2
  [MAB_alpp] -> Demux13/1
  Demux13/1 -> clm0_vs_mach_alpha_beta1/1
  [MAB_alpm] -> Demux14/1
  Demux18/3 -> cln0_vs_mach_alpha_beta2/3
  cln0_vs_mach_alpha_beta1/1 -> [cln0p]
  clm0_vs_mach_alpha_beta2/1 -> [clm0m]
  Demux18/1 -> cln0_vs_mach_alpha_beta2/1
  Demux17/2 -> cln0_vs_mach_alpha_beta1/2
  [MAB_alpm] -> Demux12/1
  cn0_vs_mach_alpha_beta2/1 -> [cn0m]
  Demux16/2 -> cy0_vs_mach_alpha_beta 2/2
  [ca0] -> aeroCoeffs/1(ca0)
  [caa] -> aeroCoeffs/2(caa)
  [cad] -> aeroCoeffs/3(cad)
  [ca0b] -> aeroCoeffs/4(ca0b)
  [cy0] -> aeroCoeffs/5(cy0)
  [cydr] -> aeroCoeffs/6(cydr)
  [cn0] -> aeroCoeffs/7(cn0)
  [cndq] -> aeroCoeffs/8(cndq)
  [cll0] -> aeroCoeffs/9(cll0)
  [cllp] -> aeroCoeffs/10(cllp)
  [clldp] -> aeroCoeffs/11(clldp)
  [clm0] -> aeroCoeffs/12(clm0)
  [clmq] -> aeroCoeffs/13(clmq)
  [clmdq] -> aeroCoeffs/14(clmdq)
  [cln0] -> aeroCoeffs/15(cln0)
  [clnr] -> aeroCoeffs/16(clnr)
  [clndr] -> aeroCoeffs/17(clndr)
  [cn0p] -> aeroCoeffs/18(cn0p)
  [cn0m] -> aeroCoeffs/19(cn0m)
  [clm0p] -> aeroCoeffs/20(clm0p)
  [clm0m] -> aeroCoeffs/21(clm0m)
  [cy0p] -> aeroCoeffs/22(cy0p)
  [cy0m] -> aeroCoeffs/23(cy0m)
  [cln0p] -> aeroCoeffs/24(cln0p)
  [cln0m] -> aeroCoeffs/25(cln0m)
  [alpp] -> aeroCoeffs/26(alpp)
  [alpm] -> aeroCoeffs/27(alpm)
  [betp] -> aeroCoeffs/28(betp)
  [betm] -> aeroCoeffs/29(betm)
  [deff] -> aeroCoeffs/30(deff)
  [dpx] -> aeroCoeffs/31(dpx)
  [dqx] -> aeroCoeffs/32(dqx)
  [drx] -> aeroCoeffs/33(drx)
  [ppx] -> aeroCoeffs/34(ppx)
  [qqx] -> aeroCoeffs/35(qqx)
  [rrx] -> aeroCoeffs/36(rrx)
  [dvbe] -> aeroCoeffs/37(dvbe)
  [pdynmc] -> aeroCoeffs/38(pdynmc)
  [mass] -> aeroCoeffs/39(mass)
  [xcg] -> aeroCoeffs/40(xcg)
  [ai11] -> aeroCoeffs/41(ai11)
  [ai33] -> aeroCoeffs/42(ai33)
  [mprop] -> aeroCoeffs/43(mprop)
  aeroCoeffs/1(ca) -> Bus Creator/1
  aeroCoeffs/2(cy) -> Bus Creator/2
  aeroCoeffs/3(cn) -> Bus Creator/3
  aeroCoeffs/4(cll) -> Bus Creator/4
  aeroCoeffs/5(clm) -> Bus Creator/5
  aeroCoeffs/6(cln) -> Bus Creator/6
  aeroCoeffs/7(dna) -> Bus Creator/7
  aeroCoeffs/8(dma) -> Bus Creator/8
  aeroCoeffs/9(dmq) -> Bus Creator/9
  aeroCoeffs/10(dmd) -> Bus Creator/10
  aeroCoeffs/11(dnd) -> Bus Creator/11
  aeroCoeffs/12(dyb) -> Bus Creator/12
  aeroCoeffs/13(dlnb) -> Bus Creator/13
  aeroCoeffs/14(dlnr) -> Bus Creator/14
  aeroCoeffs/15(dlnd) -> Bus Creator/15
  aeroCoeffs/16(dlp) -> Bus Creator/16
  aeroCoeffs/17(dld) -> Bus Creator/17
  aeroCoeffs/18(wnq) -> Bus Creator/18
  aeroCoeffs/19(wnr) -> Bus Creator/19
  aeroCoeffs/20(zetq) -> Bus Creator/20
  aeroCoeffs/21(zetr) -> Bus Creator/21
  Bus Creator/1 -> aeroBus/1
  ppx/1 -> [ppx]
  rrx/1 -> [rrx]
  dvbe/1 -> [dvbe]
  qqx/1 -> [qqx]
  thrust/1 -> [thrust]
  [thrust] -> aeroCoeffs/44(thrust)

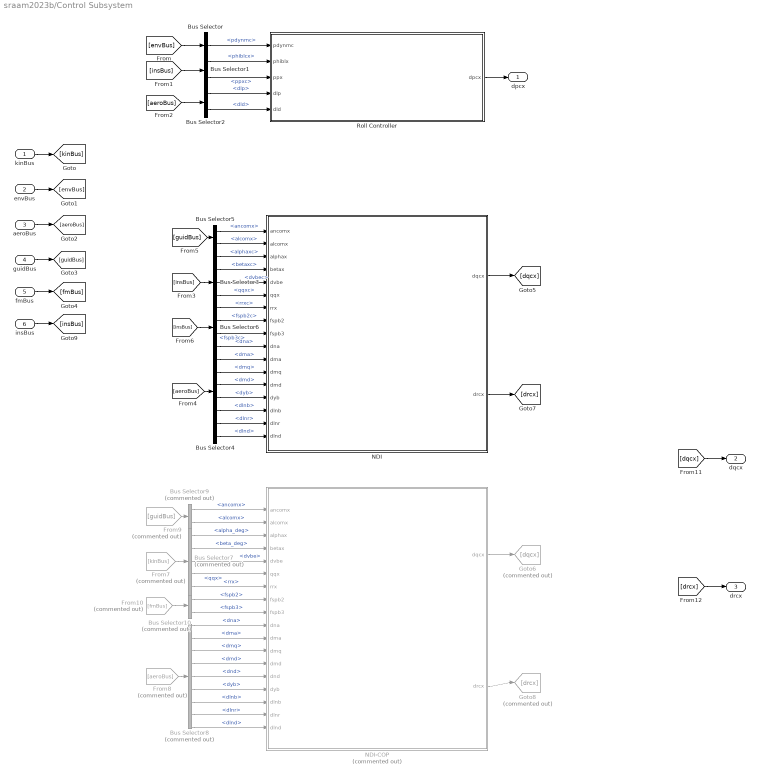
== system sraam2023b/Control Subsystem ==
  kinBus : Inport
  envBus : Inport  Port=2
  aeroBus : Inport  Port=3
  guidBus : Inport  Port=4
  fmBus : Inport  Port=5
  insBus : Inport  Port=6
  Bus Selector : BusSelector  OutputSignals=pdynmc
  Bus Selector1 : BusSelector  OutputSignals=phiblcx,ppxc
  Bus Selector10 : BusSelector  Commented=on  OutputSignals=fspb2,fspb3
  Bus Selector2 : BusSelector  OutputSignals=dlp,dld
  Bus Selector3 : BusSelector  OutputSignals=alphaxc,betaxc,dvbec,qqxc,rrxc
  Bus Selector4 : BusSelector  OutputSignals=dna,dma,dmq,dmd,dyb,dlnb,dlnr,dlnd
  Bus Selector5 : BusSelector  OutputSignals=ancomx,alcomx
  Bus Selector6 : BusSelector  OutputSignals=fspb2c,fspb3c
  Bus Selector7 : BusSelector  Commented=on  OutputSignals=alpha_deg,beta_deg,dvbe,qqx,rrx
  Bus Selector8 : BusSelector  Commented=on  OutputSignals=dna,dma,dmq,dmd,dnd,dyb,dlnb,dlnr,dlnd
  Bus Selector9 : BusSelector  Commented=on  OutputSignals=ancomx,alcomx
  From10 : From  Commented=on  GotoTag=fmBus
  From7 : From  Commented=on  GotoTag=kinBus
  From8 : From  Commented=on  GotoTag=aeroBus
  From9 : From  Commented=on  GotoTag=guidBus
  Goto6 : Goto  Commented=on  GotoTag=dqcx
  Goto8 : Goto  Commented=on  GotoTag=drcx
  NDI : MATLAB Function  TreatAsAtomicUnit=on
  NDI-COP : MATLAB Function  Commented=on  TreatAsAtomicUnit=on
  Roll Controller : MATLAB Function  TreatAsAtomicUnit=on
  dpcx : Outport
  dqcx : Outport  Port=2
  drcx : Outport  Port=3
  wires:
  kinBus/1 -> [kinBus]
  envBus/1 -> [envBus]
  aeroBus/1 -> [aeroBus]
  guidBus/1 -> [guidBus]
  fmBus/1 -> [fmBus]
  [envBus] -> Bus Selector/1
  Bus Selector/1 -> Roll Controller/1(pdynmc)  "<pdynmc>"
  [insBus] -> Bus Selector1/1
  Bus Selector1/1 -> Roll Controller/2(phiblx)  "<phiblcx>"
  Bus Selector1/2 -> Roll Controller/3(ppx)  "<ppxc>"
  [aeroBus] -> Bus Selector2/1
  Bus Selector2/1 -> Roll Controller/4(dlp)  "<dlp>"
  Bus Selector2/2 -> Roll Controller/5(dld)  "<dld>"
  Roll Controller/1(dpcx) -> dpcx/1
  [insBus] -> Bus Selector3/1
  Bus Selector3/1 -> NDI/3(alphax)  "<alphaxc>"
  Bus Selector3/2 -> NDI/4(betax)  "<betaxc>"
  Bus Selector3/3 -> NDI/5(dvbe)  "<dvbec>"
  Bus Selector3/4 -> NDI/6(qqx)  "<qqxc>"
  Bus Selector3/5 -> NDI/7(rrx)  "<rrxc>"
  [aeroBus] -> Bus Selector4/1
  Bus Selector4/1 -> NDI/10(dna)  "<dna>"
  Bus Selector4/2 -> NDI/11(dma)  "<dma>"
  Bus Selector4/3 -> NDI/12(dmq)  "<dmq>"
  Bus Selector4/4 -> NDI/13(dmd)  "<dmd>"
  Bus Selector4/5 -> NDI/14(dyb)  "<dyb>"
  Bus Selector4/6 -> NDI/15(dlnb)  "<dlnb>"
  Bus Selector4/7 -> NDI/16(dlnr)  "<dlnr>"
  Bus Selector4/8 -> NDI/17(dlnd)  "<dlnd>"
  NDI/1(dqcx) -> [dqcx]
  [guidBus] -> Bus Selector5/1
  Bus Selector5/1 -> NDI/1(ancomx)  "<ancomx>"
  Bus Selector5/2 -> NDI/2(alcomx)  "<alcomx>"
  [insBus] -> Bus Selector6/1
  Bus Selector6/1 -> NDI/8(fspb2)  "<fspb2c>"
  Bus Selector6/2 -> NDI/9(fspb3)  "<fspb3c>"
  Bus Selector8/1 -> NDI-COP/10(dna)  "<dna>"
  Bus Selector10/1 -> NDI-COP/8(fspb2)  "<fspb2>"
  Bus Selector9/1 -> NDI-COP/1(ancomx)  "<ancomx>"
  From10/1 -> Bus Selector10/1
  From9/1 -> Bus Selector9/1
  From7/1 -> Bus Selector7/1
  Bus Selector8/6 -> NDI-COP/15(dyb)  "<dyb>"
  Bus Selector10/2 -> NDI-COP/9(fspb3)  "<fspb3>"
  Bus Selector7/3 -> NDI-COP/5(dvbe)  "<dvbe>"
  Bus Selector7/5 -> NDI-COP/7(rrx)  "<rrx>"
  Bus Selector7/1 -> NDI-COP/3(alphax)  "<alpha_deg>"
  Bus Selector8/8 -> NDI-COP/17(dlnr)  "<dlnr>"
  Bus Selector7/4 -> NDI-COP/6(qqx)  "<qqx>"
  Bus Selector8/7 -> NDI-COP/16(dlnb)  "<dlnb>"
  Bus Selector7/2 -> NDI-COP/4(betax)  "<beta_deg>"
  Bus Selector8/2 -> NDI-COP/11(dma)  "<dma>"
  From8/1 -> Bus Selector8/1
  Bus Selector8/9 -> NDI-COP/18(dlnd)  "<dlnd>"
  Bus Selector9/2 -> NDI-COP/2(alcomx)  "<alcomx>"
  Bus Selector8/5 -> NDI-COP/14(dnd)  "<dnd>"
  Bus Selector8/3 -> NDI-COP/12(dmq)  "<dmq>"
  Bus Selector8/4 -> NDI-COP/13(dmd)  "<dmd>"
  NDI-COP/1(dqcx) -> Goto6/1
  NDI-COP/2(drcx) -> Goto8/1
  NDI/2(drcx) -> [drcx]
  [dqcx] -> dqcx/1
  [drcx] -> drcx/1
  insBus/1 -> [insBus]

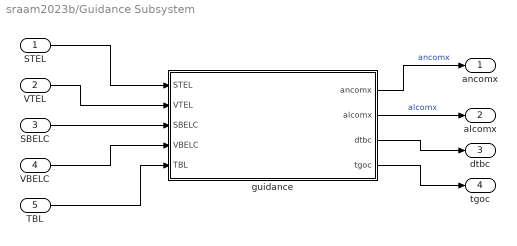
== system sraam2023b/Guidance Subsystem ==
  STEL : Inport
  VTEL : Inport  Port=2
  SBELC : Inport  Port=3
  VBELC : Inport  Port=4
  TBL : Inport  Port=5
  guidance : MATLAB Function  TreatAsAtomicUnit=on
  ancomx : Outport
  alcomx : Outport  Port=2
  dtbc : Outport  Port=3
  tgoc : Outport  Port=4
  wires:
  STEL/1 -> guidance/1(STEL)
  VTEL/1 -> guidance/2(VTEL)
  SBELC/1 -> guidance/3(SBELC)
  VBELC/1 -> guidance/4(VBELC)
  TBL/1 -> guidance/5(TBL)
  guidance/1(ancomx) -> ancomx/1  "ancomx"
  guidance/2(alcomx) -> alcomx/1  "alcomx"
  guidance/3(dtbc) -> dtbc/1
  guidance/4(tgoc) -> tgoc/1

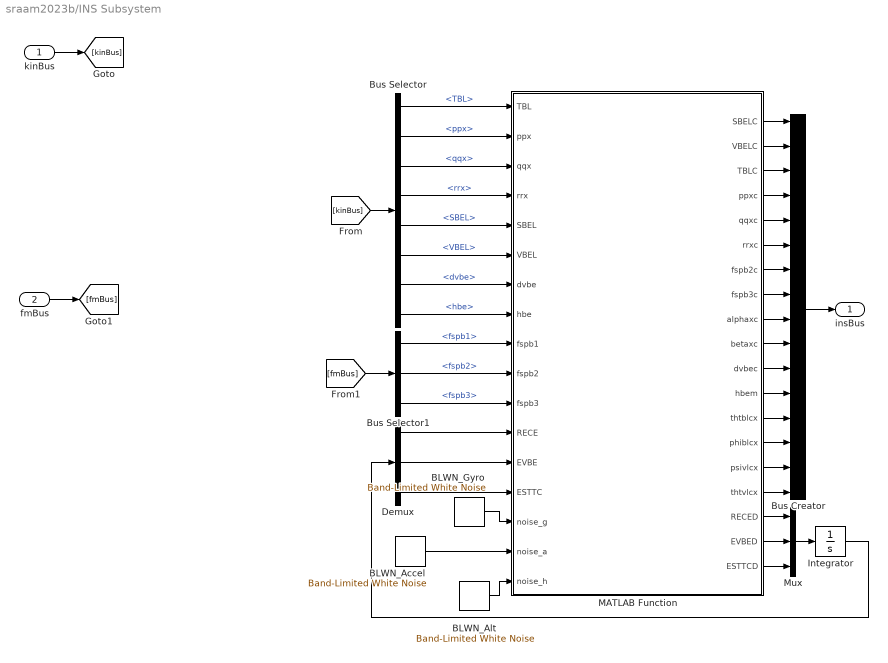
== system sraam2023b/INS Subsystem ==
  kinBus : Inport
  fmBus : Inport  Port=2
  BLWN_Accel : simulink/Sources/Band-Limited White Noise  Cov=INS_NOISE_PWR_A * [1; 1; 1]  Ts=DT  seed=[23341]
  BLWN_Alt : simulink/Sources/Band-Limited White Noise  Cov=INS_NOISE_PWR_H  Ts=DT  seed=[23341]
  BLWN_Gyro : simulink/Sources/Band-Limited White Noise  Cov=INS_NOISE_PWR_G * [1; 1; 1]  Ts=DT  seed=[23341]
  Bus Creator : BusCreator  Inputs=16
  Bus Selector : BusSelector  OutputSignals=TBL,ppx,qqx,rrx,SBEL,VBEL,dvbe,hbe
  Bus Selector1 : BusSelector  OutputSignals=fspb1,fspb2,fspb3
  Demux : Demux  Outputs=3
  Integrator : Integrator  InitialCondition=zeros(9, 1)
  MATLAB Function : MATLAB Function  TreatAsAtomicUnit=on
  Mux : Mux  Inputs=3
  insBus : Outport
  wires:
  kinBus/1 -> [kinBus]
  fmBus/1 -> [fmBus]
  Mux/1 -> Integrator/1
  Integrator/1 -> Demux/1
  Demux/1 -> MATLAB Function/12(RECE)
  Demux/2 -> MATLAB Function/13(EVBE)
  Demux/3 -> MATLAB Function/14(ESTTC)
  [kinBus] -> Bus Selector/1
  Bus Selector/1 -> MATLAB Function/1(TBL)  "<TBL>"
  Bus Selector/2 -> MATLAB Function/2(ppx)  "<ppx>"
  Bus Selector/3 -> MATLAB Function/3(qqx)  "<qqx>"
  Bus Selector/4 -> MATLAB Function/4(rrx)  "<rrx>"
  Bus Selector/5 -> MATLAB Function/5(SBEL)  "<SBEL>"
  Bus Selector/6 -> MATLAB Function/6(VBEL)  "<VBEL>"
  Bus Selector/7 -> MATLAB Function/7(dvbe)  "<dvbe>"
  Bus Selector/8 -> MATLAB Function/8(hbe)  "<hbe>"
  [fmBus] -> Bus Selector1/1
  Bus Selector1/1 -> MATLAB Function/9(fspb1)  "<fspb1>"
  Bus Selector1/2 -> MATLAB Function/10(fspb2)  "<fspb2>"
  Bus Selector1/3 -> MATLAB Function/11(fspb3)  "<fspb3>"
  MATLAB Function/19(ESTTCD) -> Mux/3
  MATLAB Function/18(EVBED) -> Mux/2
  MATLAB Function/17(RECED) -> Mux/1
  BLWN_Gyro/1 -> MATLAB Function/15(noise_g)
  BLWN_Accel/1 -> MATLAB Function/16(noise_a)
  BLWN_Alt/1 -> MATLAB Function/17(noise_h)
  MATLAB Function/1(SBELC) -> Bus Creator/1
  MATLAB Function/2(VBELC) -> Bus Creator/2
  MATLAB Function/3(TBLC) -> Bus Creator/3
  MATLAB Function/4(ppxc) -> Bus Creator/4
  MATLAB Function/5(qqxc) -> Bus Creator/5
  MATLAB Function/6(rrxc) -> Bus Creator/6
  MATLAB Function/7(fspb2c) -> Bus Creator/7
  MATLAB Function/8(fspb3c) -> Bus Creator/8
  MATLAB Function/9(alphaxc) -> Bus Creator/9
  MATLAB Function/10(betaxc) -> Bus Creator/10
  MATLAB Function/11(dvbec) -> Bus Creator/11
  MATLAB Function/12(hbem) -> Bus Creator/12
  MATLAB Function/13(thtblcx) -> Bus Creator/13
  MATLAB Function/14(phiblcx) -> Bus Creator/14
  MATLAB Function/15(psivlcx) -> Bus Creator/15
  MATLAB Function/16(thtvlcx) -> Bus Creator/16
  Bus Creator/1 -> insBus/1

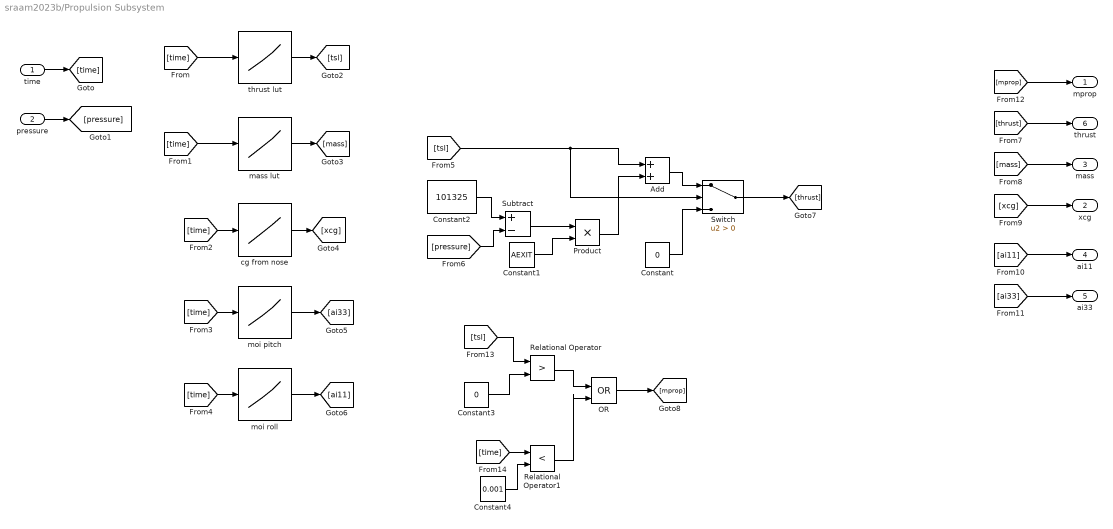
== system sraam2023b/Propulsion Subsystem ==
  time : Inport
  pressure : Inport  Port=2
  Add : Sum
  Constant : Constant  Value=0
  Constant1 : Constant  Value=AEXIT
  Constant2 : Constant  Value=101325
  Constant3 : Constant  Value=0
  Constant4 : Constant  Value=0.001
  OR : Logic  Operator=OR  IconShape=distinctive  AllPortsSameDT=off  OutDataTypeStr=boolean
  Product : Product
  Relational Operator : RelationalOperator  Operator=>  OutDataTypeStr=boolean  RndMeth=Simplest  InputSameDT=off
  Relational Operator1 : RelationalOperator  Operator=<  OutDataTypeStr=boolean  RndMeth=Simplest  InputSameDT=off
  Subtract : Sum  Inputs=+-
  Switch : Switch  Criteria=u2 > Threshold  SaturateOnIntegerOverflow=off  InputSameDT=off
  cg from nose : Lookup_n-D  NumberOfTableDimensions=1  BreakpointsForDimension1=prop_cg_t  Table=prop_cg_v  ExtrapMethod=Clip  UseLastTableValue=on  InternalRulePriority=Speed  RndMeth=Simplest
  mass lut : Lookup_n-D  NumberOfTableDimensions=1  BreakpointsForDimension1=prop_mass_t  Table=prop_mass_v  ExtrapMethod=Clip  UseLastTableValue=on  InternalRulePriority=Speed  RndMeth=Simplest
  moi pitch : Lookup_n-D  NumberOfTableDimensions=1  BreakpointsForDimension1=prop_moipitch_t  Table=prop_moipitch_v  ExtrapMethod=Clip  UseLastTableValue=on  InternalRulePriority=Speed  RndMeth=Simplest
  moi roll : Lookup_n-D  NumberOfTableDimensions=1  BreakpointsForDimension1=prop_moiroll_t  Table=prop_moiroll_v  ExtrapMethod=Clip  UseLastTableValue=on  InternalRulePriority=Speed  RndMeth=Simplest
  thrust lut : Lookup_n-D  NumberOfTableDimensions=1  BreakpointsForDimension1=prop_thrust_t  Table=prop_thrust_v  ExtrapMethod=Clip  UseLastTableValue=on  InternalRulePriority=Speed  RndMeth=Simplest
  mprop : Outport
  xcg : Outport  Port=2
  mass : Outport  Port=3
  ai11 : Outport  Port=4
  ai33 : Outport  Port=5
  thrust : Outport  Port=6
  wires:
  Product/1 -> Add/2
  moi roll/1 -> [ai11]
  [pressure] -> Subtract/2
  [time] -> thrust lut/1
  [mass] -> mass/1
  [tsl] -> Relational Operator/1
  [xcg] -> xcg/1
  [mprop] -> mprop/1
  Constant1/1 -> Product/2
  pressure/1 -> [pressure]
  [ai11] -> ai11/1
  Subtract/1 -> Product/1
  moi pitch/1 -> [ai33]
  [time] -> mass lut/1
  cg from nose/1 -> [xcg]
  [thrust] -> thrust/1
  [tsl] -> Add/1, Switch/2
  time/1 -> [time]
  mass lut/1 -> [mass]
  thrust lut/1 -> [tsl]
  [ai33] -> ai33/1
  Constant2/1 -> Subtract/1
  [time] -> moi pitch/1
  [time] -> cg from nose/1
  [time] -> moi roll/1
  Constant3/1 -> Relational Operator/2
  Add/1 -> Switch/1
  Switch/1 -> [thrust]
  Constant/1 -> Switch/3
  Relational Operator/1 -> OR/1
  OR/1 -> [mprop]
  [time] -> Relational Operator1/1
  Constant4/1 -> Relational Operator1/2
  Relational Operator1/1 -> OR/2

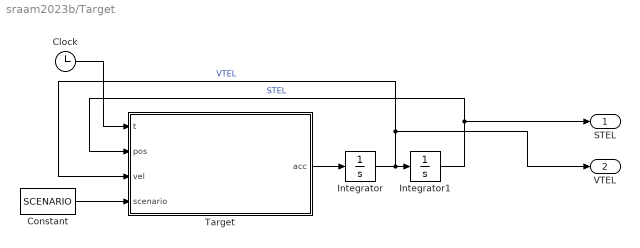
== system sraam2023b/Target ==
  Clock : Clock
  Constant : Constant  Value=SCENARIO
  Integrator : Integrator  InitialCondition=TGET_VEL_IC
  Integrator1 : Integrator  InitialCondition=TGET_POS_IC
  Target : MATLAB Function  TreatAsAtomicUnit=on
  STEL : Outport
  VTEL : Outport  Port=2
  wires:
  Constant/1 -> Target/4(scenario)
  Target/1(acc) -> Integrator/1
  Integrator/1 -> VTEL/1, Target/3(vel), Integrator1/1  "VTEL"
  Integrator1/1 -> Target/2(pos), STEL/1  "STEL"
  Clock/1 -> Target/1(t)

== matlab function sraam2023b/Environment Subsystem ==
  data: hbe input; rho output; dvbe input; press output; tempk output; vsound output; grav output; mach output; pdynmc output
function [rho, press, tempk, vsound, grav, mach, pdynmc] = environment(hbe, dvbe)
%ENVIRONMENT  US 1976 Standart Atmosfer + yerçekimi + Mach + dinamik basınç.
% Kaynak: missile/environment.py
%#codegen

% Fiziksel sabitler (environment.py:4-8)
REARTH     = 6.3781e6;
G_CONST    = 6.674e-11;
EARTH_MASS = 5.9722e24;
R_AIR      = 287.058;
G0         = 9.80665;

h = max(hbe, 0.0);

% ── US76 Standart Atmosfer (environment.py:18-57) ────────────────────────────
if h <= 11000.0
    T = 288.15 - 6.5e-3 * h;
    P = 101325.0 * (T / 288.15)^5.25588;

elseif h <= 20000.0
    T = 216.65;
    P = 22632.1 * exp(-G0 / (R_AIR * T) * (h - 11000.0));

elseif h <= 32000.0
    T = 216.65 + 1.0e-3 * (h - 20000.0);
    P = 5474.89 * (T / 216.65)^(-G0 / (R_AIR * 1.0e-3));

elseif h <= 47000.0
    T = 228.65 + 2.8e-3 * (h - 32000.0);
    P = 868.019 * (T / 228.65)^(-G0 / (R_AIR * 2.8e-3));

elseif h <= 51000.0
    T = 270.65;
    P = 110.906 * exp(-G0 / (R_AIR * T) * (h - 47000.0));

elseif h <= 71000.0
    T = 270.65 - 2.8e-3 * (h - 51000.0);
    P = 66.9389 * (T / 270.65)^(G0 / (R_AIR * 2.8e-3));

else
    T = 214.65 - 2.0e-3 * (h - 71000.0);
    P = 3.95642 * (T / 214.65)^(G0 / (R_AIR * 2.0e-3));
end

rho    = P / (R_AIR * T);
press  = P;
tempk  = T;

% ── Ses hızı, Mach, dinamik basınç ───────────────────────────────────────────
vsound = sqrt(1.4 * R_AIR * T);
mach   = abs(dvbe / vsound);
pdynmc = 0.5 * rho * dvbe * dvbe;

% ── Yerçekimi (ters kare kanunu) ─────────────────────────────────────────────
rad  = REARTH + hbe;
grav = G_CONST * EARTH_MASS / (rad * rad);
end

== matlab function sraam2023b/Aerodynamics Subsystem/aeroCoeffs ==
  data: ca0 input; ca output; caa input; cad input; ca0b input; cy0 input; cydr input; cn0 input; cndq input; cll0 input; cllp input; clldp input; clm0 input; clmq input; clmdq input; cln0 input; clnr input; clndr input; cn0p input; cn0m input; clm0p input; clm0m input; cy0p input; cy0m input; cln0p input; cln0m input; alpp input; alpm input; betp input; betm input; deff input; dpx input; dqx input; drx input; ppx input; qqx input; rrx input; dvbe input; pdynmc input; mass input; xcg input; ai11 input; ai33 input; mprop input; thrust input; cy output; cn output; cll output; clm output; cln output; dna output; dma output; dmq output; dmd output; dnd output; dyb output; dlnb output; dlnr output; dlnd output; dlp output; dld output; wnq output; wnr output; zetq output; zetr output; REFL parameter; REFA parameter; XCG_REF parameter
function [ca, cy, cn, cll, clm, cln, ...
          dna, dma, dmq, dmd, dnd, ...
          dyb, dlnb, dlnr, dlnd, dlp, dld, ...
          wnq, wnr, zetq, zetr] = ...
    aero_coeff( ...
        ca0, caa, cad, ca0b, ...
        cy0, cydr, ...
        cn0, cndq, ...
        cll0, cllp, clldp, ...
        clm0, clmq, clmdq, ...
        cln0, clnr, clndr, ...
        cn0p, cn0m, clm0p, clm0m, ...
        cy0p, cy0m, cln0p, cln0m, ...
        alpp, alpm, betp, betm, ...
        deff, ...
        dpx, dqx, drx, ppx, qqx, rrx, ...
        dvbe, pdynmc, mass, xcg, ai11, ai33, mprop, thrust, REFL, REFA, XCG_REF)
%AERO_COEFF  Katsayılar + boyutsal türevler — tüm girişler LUT çıkışı skalardır.
% Kaynak: missile/aerodynamics.py
%#codegen

SMALL  = 1e-7;
DEG    = 180.0 / pi;
RAD    = pi / 180.0;

% Workspace parametreleri (Symbols → Parameter)
refl   = REFL;
refa   = REFA;
xcgref = XCG_REF;

% ── Eksenel kuvvet ────────────────────────────────────────────────────────────
ca  = ca0 + caa + cad * deff^2;
if mprop > 0;  ca = ca + ca0b;  end

% ── Yan ve normal kuvvetler ───────────────────────────────────────────────────
cy  = cy0  + cydr  * drx;
cn  = cn0  + cndq  * dqx;

% ── Momentler ─────────────────────────────────────────────────────────────────
cll = cllp * RAD * ppx * refl / (2.0*dvbe) + cll0 + clldp * dpx;
clm = clm0 + clmq * RAD * qqx * refl / (2.0*dvbe) + clmdq * dqx ...
      - cn/refl * (xcgref - xcg);
cln = cln0 + clnr * RAD * rrx * refl / (2.0*dvbe) + clndr * drx ...
      - cy/refl * (xcgref - xcg);

% ── ND türevler ───────────────────────────────────────────────────────────────
da  = alpp - alpm;
cna  = DEG * (cn0p  - cn0m)  / (da + SMALL);
clma = DEG * (clm0p - clm0m) / (da + SMALL) - cna/refl*(xcgref-xcg);

db   = betp - betm;
cyb  = DEG * (cy0p  - cy0m)  / (db + SMALL);
clnb = DEG * (cln0p - cln0m) / (db + SMALL) - cyb/refl*(xcgref-xcg);

% ── Boyutsal türevler ─────────────────────────────────────────────────────────
dna  = (pdynmc*refa/mass)                           * cna;
dma  = (pdynmc*refa*refl/ai33)                      * clma;
dmq  = DEG*(pdynmc*refa*refl/ai33)*(refl/(2*dvbe))  * clmq * RAD;
dmd  = DEG*(pdynmc*refa*refl/ai33)                  * clmdq;
dnd  = (pdynmc*refa/mass)                           * cndq;
dyb  = (pdynmc*refa/mass)                           * cyb;
dlnb = (pdynmc*refa*refl/ai33)                      * clnb;
dlnr = DEG*(pdynmc*refa*refl/ai33)*(refl/(2*dvbe))  * clnr * RAD;
dlnd = DEG*(pdynmc*refa*refl/ai33)                  * clndr;
dlp  = DEG*(pdynmc*refa*refl/ai11)*(refl/(2*dvbe))  * cllp * RAD;
dld  = DEG*(pdynmc*refa*refl/ai11)                  * clldp;

% ── Dinamik kökler ────────────────────────────────────────────────────────────
a11q = dmq;  a12q = dma/(dna+SMALL);
a21q = dna;  a22q = -dna/(dvbe+SMALL);
argq = (a11q+a22q)^2 - 4*(a11q*a22q - a12q*a21q);
if argq >= 0;  wnq=0.0; zetq=0.0;
else;  wnq=sqrt(-(argq)/4.0 + ((a11q+a22q)/2)^2 - (a11q+a22q)^2/4);
       wnq=sqrt(max(a11q*a22q - a12q*a21q, 0));
       zetq=-(a11q+a22q)/(2*max(wnq,SMALL)); end

a11r = dlnr;  a12r = dlnb/(dyb+SMALL);
a21r = -dyb;  a22r = dyb/(dvbe+SMALL);
argr = (a11r+a22r)^2 - 4*(a11r*a22r - a12r*a21r);
if argr >= 0;  wnr=0.0; zetr=0.0;
else;  wnr=sqrt(max(a11r*a22r - a12r*a21r, 0));
       zetr=-(a11r+a22r)/(2*max(wnr,SMALL)); end

end

== matlab function sraam2023b/Forces and Moments ==
  data: ca input; FAPB output; cy input; cn input; cll input; clm input; cln input; thrust input; pdynmc input; FMB output; fspb1 output; fspb2 output; fspb3 output; mass input; REFA parameter; REFL parameter
function [FAPB, FMB, fspb1, fspb2, fspb3] = forces(ca, cy, cn, cll, clm, cln, thrust, pdynmc, mass, REFA, REFL)
%FORCES  Toplam kuvvet ve moment vektörleri — gövde ekseni.
% Kaynak: missile/forces.py
%#codegen

refa = REFA;   % workspace parametresi
refl = REFL;   % workspace parametresi

% Aerodinamik kuvvetler + itki (forces.py:33-45)
FAPB = [-pdynmc * refa * ca + thrust;
         pdynmc * refa * cy;
        -pdynmc * refa * cn];

% Aerodinamik momentler (forces.py:51-55)
FMB = pdynmc * refa * refl * [cll; clm; cln];

% Spesifik kuvvet (newton.py: FSPB = FAPB/mass) — control_ndi için
fspb1 = FAPB(1) / mass;
fspb2 = FAPB(2) / mass;
fspb3 = FAPB(3) / mass;
end

== matlab function sraam2023b/Actuator Subsystem/actuator_deriv ==
  data: x_act input; xdot output; dpcx input; dqcx input; drcx input; dpx output; dqx output; drx output; del1 output; del2 output; del3 output; del4 output; WNACT parameter; ZETACT parameter; DLIMX parameter; DDLIMX parameter
function [xdot, dpx, dqx, drx, del1, del2, del3, del4] = ...
         actuator_deriv(x_act, dpcx, dqcx, drcx, WNACT, ZETACT, DLIMX, DDLIMX)
%ACTUATOR_DERIV  2. mertebe fin aktüatör dinamikleri.
% Kaynak: missile/actuator.py — actuator_scnd()
%
% Durum vektörü x_act [8x1]:
%   x_act(1:4)  = [del1, del2, del3, del4]   fin konumları - deg
%   x_act(5:8)  = [del1d, del2d, del3d, del4d] fin hızları - deg/s
%
% Girişler: dpcx, dqcx, drcx — kontrolcü komutları - deg
% Çıkışlar: xdot[8], dpx, dqx, drx — gerçek defleksiyonlar - deg
%#codegen

wnact  = WNACT;    % workspace parametresi - rad/s
zetact = ZETACT;   % workspace parametresi
dlimx  = DLIMX;    % konum sınırı - deg
ddlimx = DDLIMX;   % hız sınırı - deg/s

wn2 = wnact * wnact;

% ── Komut karışımı (actuator.py:63-66) ───────────────────────────────────────
delcx1 = -dpcx + dqcx - drcx;
delcx2 = -dpcx + dqcx + drcx;
delcx3 = +dpcx + dqcx - drcx;
delcx4 = +dpcx + dqcx + drcx;

delcx = [delcx1; delcx2; delcx3; delcx4];

% ── Durum ─────────────────────────────────────────────────────────────────────
del  = x_act(1:4);    % konum - deg
deld = x_act(5:8);    % hız - deg/s

% ── 2. mertebe ODE türevleri (actuator.py:134) ───────────────────────────────
deldd = wn2 * (delcx - del) - 2.0 * zetact * wnact * deld;

% ── Hız sınırlayıcı (actuator.py:141-142) ────────────────────────────────────
% Not: Simulink integratörü sınırla → Rate Limiter bloğuyla veya
%      türevi burada klip yap (yaklaşık)
deld_lim = max(min(deld, ddlimx), -ddlimx);

% ── Türev vektörü ─────────────────────────────────────────────────────────────
% dkonum/dt = hız (sınırlı)
% dhız/dt   = ikinci türev
xdot = [deld_lim; deldd];

% ── Konum sınırlayıcı (çıkış klibi) ─────────────────────────────────────────
del_out = max(min(del, dlimx), -dlimx);

% ── Geri dönüşüm: fin defleksiyon → roll/pitch/yaw (actuator.py:87-89) ───────
dpx = (-del_out(1) - del_out(2) + del_out(3) + del_out(4)) / 4.0;
dqx = (+del_out(1) + del_out(2) + del_out(3) + del_out(4)) / 4.0;
drx = (-del_out(1) + del_out(2) - del_out(3) + del_out(4)) / 4.0;

del1 = del_out(1);
del2 = del_out(2);
del3 = del_out(3);
del4 = del_out(4);
end

== matlab function sraam2023b/Control Subsystem/Roll Controller ==
  data: pdynmc input; dpcx output; phiblx input; ppx input; dlp input; dld input; ZRCL parameter; FACT_WRCL parameter; DPLIMX parameter
function dpcx = control_roll(pdynmc, phiblx, ppx, dlp, dld, ZRCL, FACT_WRCL, DPLIMX)
% ppx: roll hızı deg/s (kinBus'tan direkt gelir)
%CONTROL_ROLL  Yuvarlanma pozisyon kontrolcüsü.
% Kaynak: missile/control.py — control_roll()
%#codegen

RAD   = pi / 180.0;
DEG   = 180.0 / pi;
SMALL = 1e-7;

zrcl     = ZRCL;
factwrcl = FACT_WRCL;
dplimx   = DPLIMX;
phicomx  = 0.0;   % banka açısı komutu — Guidance eklenince değişir

% Değişken roll bant genişliği
wrcl  = (0.00024 * pdynmc + 10.0) * (1.0 + factwrcl);

% Kazançlar
dld_s = dld; if abs(dld_s) < SMALL; dld_s = SMALL; end
gkp   = (2.0 * zrcl * wrcl + dlp) / dld_s;
gkphi = wrcl * wrcl / dld_s;

% Roll pozisyon komutu (pp = ppx*RAD, gkp pp üzerinden çalışır)
pp   = ppx * RAD;
dpc  = gkphi * (phicomx - phiblx) * RAD - gkp * pp;
dpcx = max(min(dpc * DEG, dplimx), -dplimx);
end
